simulink library "create_mdot"  (Simulink 8.2)
settings: Solver=ode45  StartTime=0.0  StopTime=10.0  RelTol=1e-3
libraries: simulink x4
settings Model: Creator=lena.frank  LastModifiedBy=drhf

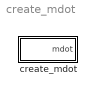
== system create_mdot ==
  create_mdot : Subsystem  mask(Create Massflow Profile){}
      settings: OpenFcn=CarnotCallbacks_create_mdot('initialize',gcb);
      mask Help: web(fullfile(path_carnot('help'),'create_mdot.html'),'-helpbrowser')

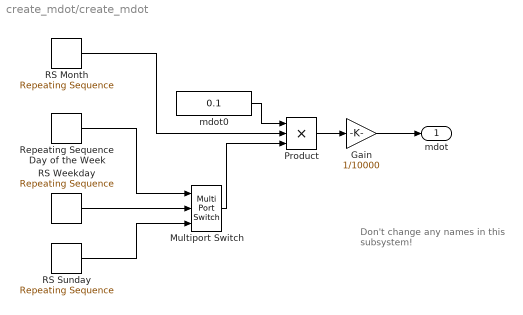
== system create_mdot/create_mdot ==
  note: Don't change any names
      | in this subsystem!
  Gain : Gain  Gain=1/10000  SaturateOnIntegerOverflow=on  OutDataTypeStr=Inherit: Same as input  ParamDataTypeStr=Inherit: Same as input
  Multiport Switch : MultiPortSwitch  Inputs=2  SaturateOnIntegerOverflow=on  InputSameDT=on
  Product : Product  Inputs=3  SaturateOnIntegerOverflow=on  InputSameDT=on  OutDataTypeStr=Inherit: Same as first input
  RS Month : simulink/Sources/Repeating Sequence  rep_seq_t=[0 2678399 2678399 5097599 5097599 7775999 7775999 10367999 10367999 13046399 13046399 15638399 15638399 18316799 18316799 20995199 20995199 23587199 23587199 26265599 26265599 28857599 28857599 31536000]  rep_seq_y=[99 99 97 97 100 100 100 100 103 103 105 105 109 109 112 112 108 108 105 105 101 101 100 100]
  RS Sunday : simulink/Sources/Repeating Sequence  rep_seq_t="100*[0 18 18 36 36 54 54 72 72 90 90 108 108 126 126 144 144 162 162 180 180 198 198 216 216 234 234 252 252 270 270 288 288 306 306 324 324 342 342 360 360 378 378 396 396 414 414 432 432 450 450 468 468 486 486 504 504 522 522 540 540 558 558 576 576 594 594 612 612 630 630 648 648 666 666 684 684 702 702 720 720 738 738 756 756 774 774 792 792 810 810 828 828 846 846  864]"  rep_seq_y=[0 0 0 0 0.5 0.5 0.5 0.5 0.5 0.5 0.5 0.5 1 1 1 1 1 1 1 1 1 1 1 1 1 1 2 2 2 2 3 3 2 2 2 2 2 2 2 2 3 3 2 2 2 2 2 2 3 3 3 3 3 3 3 3 3 3 2 2 2 2 1 1 1 1 2 2 2 2 3 3 3 3 3 3 3 3 2 2 2 2 2 2 2 2 2 2 1 1 1 1 1 1 1 1]
  RS Weekday : simulink/Sources/Repeating Sequence  rep_seq_t="100*[0 18 18 36 36 54 54 72 72 90 90 108 108 126 126 144 144 162 162 180 180 198 198 216 216 234 234 252 252 270 270 288 288 306 306 324 324 342 342 360 360 378 378 396 396 414 414 432 432 450 450 468 468 486 486 504 504 522 522 540 540 558 558 576 576 594 594 612 612 630 630 648 648 666 666 684 684 702 702 720 720 738 738 756 756 774 774 792 792 810 810 828 828 846 846  864]"  rep_seq_y=[0.5 0.5 0.5 0.5 0.5 0.5 0.5 0.5 0.5 0.5 0.5 0.5 1 1 1 1 1 1 1 1 2 2 2 2 3 3 3 3 5 5 5 5 5 5 5 5 4 4 4 4 3 3 2 2 2 2 2 2 3 3 3 3 4 4 4 4 3 3 2 2 2 2 1 1 1 1 2 2 2 2 3 3 3 3 3 3 3 3 2 2 2 2 2 2 2 2 2 2 1 1 1 1 1 1 1 1]
  Repeating Sequence Day of the Week : simulink/Sources/Repeating Sequence  rep_seq_t=[0 5*24*3600 5*24*3600 7*24*3600]  rep_seq_y=[1 1 2 2]
  mdot0 : Constant  Value=0.1
  mdot : Outport
  wires:
  Repeating Sequence Day of the Week/1 -> Multiport Switch/1
  RS Sunday/1 -> Multiport Switch/3
  Multiport Switch/1 -> Product/3
  mdot0/1 -> Product/1
  Product/1 -> Gain/1
  Gain/1 -> mdot/1
  RS Weekday/1 -> Multiport Switch/2
  RS Month/1 -> Product/2
